simulink model "DC_Motor_WhiteBox"  (R2023b)
settings: Solver=VariableStepAuto  StartTime=0.0  StopTime=10.0  RelTol=1e-3
libraries: fl_lib x5, nesl_utility x4, ee_lib x2
settings Model: Creator=Lucas  LastModifiedBy=Lucas

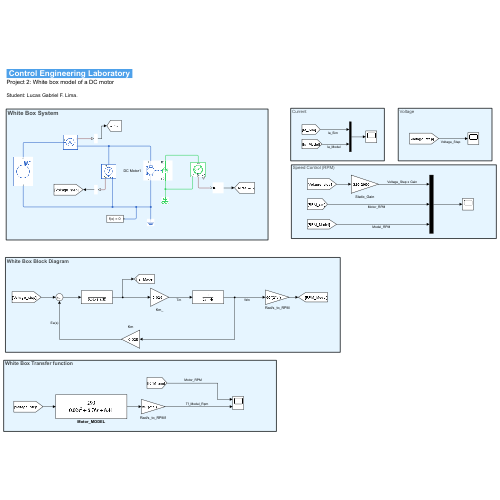
[thumbnail: Simulink's stored preview of the top-level diagram]
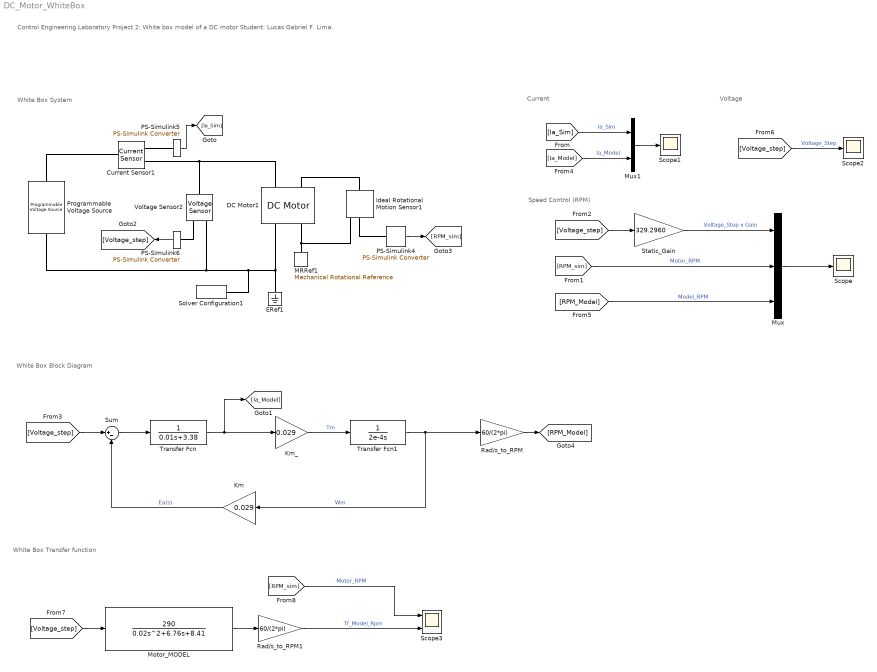
== system DC_Motor_WhiteBox ==
  note: White Box Block Diagram
  note: Speed Control (RPM)
  note: Current
  note: White Box System
  note: White Box Transfer function
  note: Control Engineering Laboratory
      | Project 2: White box model of a DC motor
      |
      | Student: Lucas Gabriel F. Lima.
  note: Voltage
  Current Sensor1 : fl_lib/Electrical/Electrical Sensors/Current Sensor
  DC Motor1 : ee_lib/Electromechanical/Brushed Motors/DC Motor  field_option=ee.enum.field_option.pm  Rf=100 Ohm  Lf=1 H  Laf=0.15 H  If0=0 A  parameterization=ee.enum.dcparam_option.circuit_param  Ra=3.38 Ohm  La=0.01 H  emf_or_torque=ee.enum.emf_or_torque.kv  Kv=0.029 V/(rad/s)  Ki=6.876e-04 N*m/A  T_stall=0.1 N*m  w_max=4000 rpm  w_rated=2500 rpm  P_rated=10 W  V_rated=12 V  lam_param=ee.enum.lam_param.damping  i_noload=0 A  V_i_noload=1.5 V  J=0.0002 kg*m^2  lam=0 N*m/(rad/s)  speed0=0 rpm  enable_fault_armature=simscape.enum.onoff.off  rev_faulted=1 / 3  G_faulted_armature=1e-5 S  fault_trigger_armature=ee.enum.faults.faultTrigger.temporal  t_fault_armature=1 s  max_permissible_current_armature=inf A  t_fail_on_current_armature=1 s  enable_fault_field=simscape.enum.onoff.off  G_faulted_field=1e-5 S  fault_trigger_field=ee.enum.faults.faultTrigger.temporal  t_fault_field=1 s  max_permissible_current_field=inf A  t_fail_on_current_field=1 s  fault_action=simscape.enum.assert.action.none  alpha=3.93e-3 1/K  Tmeas=25 degC  thermal_mass=100 J/K  initial_temperature=25 degC
  ERef1 : fl_lib/Electrical/Electrical Elements/Electrical Reference
  Ideal Rotational Motion Sensor1 : fl_lib/Mechanical/Mechanical Sensors/Ideal Rotational Motion Sensor  reference=foundation.enum.MeasurementReference.difference  acceleration_port=false  velocity_port=true  position_port=true  wrap_angle=simscape.enum.onoff.off  offset=0 deg
  Km : Gain  Gain=0.029
  Km_ : Gain  Gain=0.029
  MRRef1 : fl_lib/Mechanical/Rotational Elements/Mechanical Rotational Reference
  Motor_MODEL : TransferFcn  Numerator=[290]  Denominator=[0.02 6.76 8.41]
  Mux : Mux  Inputs=3
  Mux1 : Mux  Inputs=2
  PS-Simulink4 : nesl_utility/PS-Simulink Converter  PhysicalDomain=network_engine_domain  SubClassName=ps_output  LeftPortType=input  RightPortType=output  PseudoPeriodic=off  Frequencies=[]  VectorFormat=1-D array  Unit=rpm  AffineConversion=off
  PS-Simulink5 : nesl_utility/PS-Simulink Converter  PhysicalDomain=network_engine_domain  SubClassName=ps_output  LeftPortType=input  RightPortType=output  PseudoPeriodic=off  Frequencies=[]  VectorFormat=1-D array  Unit=A  AffineConversion=off
  PS-Simulink6 : nesl_utility/PS-Simulink Converter  PhysicalDomain=network_engine_domain  SubClassName=ps_output  LeftPortType=input  RightPortType=output  PseudoPeriodic=off  Frequencies=[]  VectorFormat=1-D array  Unit=V  AffineConversion=off
  Programmable Voltage Source : ee_lib/Sources/Programmable Voltage Source  magnitude_type=ee.enum.timechanging.constant  ac_magnitude=0 V  magn_ramp=1 V/s  magn_step=1 V  magn_modu_magn=1 V  magn_modu_freq=1 Hz  magn_t1=1 s  magn_t2=2 s  frequency_type=ee.enum.timechanging.constant  ac_frequency=60 Hz  freq_ramp=1 Hz/s  freq_step=1 Hz  freq_modu_magn=1 Hz  freq_modu_freq=1 Hz  freq_t1=1 s  freq_t2=2 s  phase_type=ee.enum.timechanging.constant  ac_shift=0 deg  phase_ramp=1 deg/s  phase_step=1 deg  phase_modu_magn=1 deg  phase_modu_freq=1 Hz  phase_t1=1 s  phase_t2=2 s  dc_type=ee.enum.timechanging.step  dc_voltage=0 V  dc_ramp=1 V/s  dc_step=1 V  dc_modu_magn=1 V  dc_modu_freq=1 Hz  dc_t1=1 s  dc_t2=10 s  harmonic_option=0  harmonic_orders=[5, 7, 11, 13]  harmonic_ratios=[.1, .1, .1, .1]  harmonic_shifts=[0, 0, 0, 0] deg  harmonic_t1=-inf s  harmonic_t2=inf s  noise_mode=0  PSD=0 V^2/Hz  repeatability=1  auto_seed=0  user_seed=0  sample_time=1e-3 s  i_specify=off  i_priority=None  i=0 A  i_nominal_specify=off  i_nominal_unit=A  i_nominal_value=1  v_specify=off  v_priority=None  v=0 V  v_nominal_specify=off  v_nominal_unit=V  v_nominal_value=1
      settings: InternalSimscapePortConfiguration="{\"Bottom\":[],\"Left\":[{\"id\":\"p\",\"label\":\"+\",\"type\":\"foundation.electrical.electrical\"}],\"Right\":[{\"id\":\"n\",\"label\":\"-\",\"type\":\"foundation.electrical.electrical\"}],\"Top\":[]}"
  Rad/s_to_RPM : Gain  Gain=60/(2*pi)
  Rad/s_to_RPM1 : Gain  Gain=60/(2*pi)
  Scope : Scope
  Scope1 : Scope
  Scope2 : Scope
  Scope3 : Scope  NumInputPorts=2
  Solver Configuration1 : nesl_utility/Solver Configuration  PhysicalDomain=network_engine_domain  SubClassName=solver  LeftPortType=input  RightPortType=generic  Tones=[]  Harmonics=[]  SimulateNoise=off  Profile=off  UseLocalSampling=off  EnableSwitchedLinearOptims=on  FrequencyDomain=off  UseCCode=off  RelTol=0.001  AbsTol=1e-06  MinStep=1e-09  ToWorkspace=off  RevertToSquareIcSolve=off  NumHomotopyIterations=100  PhasorMode=off  PhasorModeNumHarmonics=1  ConsistencySolver=NEWTON_FTOL  IndexReductionMethod=DerivativeReplacement  DoDC=off  ResidualTolerance=1e-9  ConsistencyTolSource=GLOBAL  ConsistencyAbsTol=0.001  ConsistencyRelTol=0.001  ConsistencyTolFactor=0.001  UseLocalSolver=off  LocalSolverChoice=NE_BACKWARD_EULER_ADVANCER  ResolveIndetEquations=on  FunctionEvalNumThread=1  LocalSolverSampleTime=5e-6  DoFixedCost=off  MaxNonlinIter=4  MaxModeIter=2  ComputeImpulses=off  ImpulseIterations=2  LinearAlgebra=auto  LinearAlgebraNumThread=0  EquationFormulation=NE_TIME_EF  DelaysMemoryBudget=1024  AutomaticFiltering=on  FilteringTimeConstant=0.001  PartitionStorageMethod=AS_NEEDED  PartitionMemoryBudget=1024  PartitionMethod=FAST  MultibodyUseLocalSolver=off  MultibodyLocalSolverChoice=ODE1  MultibodyLocalSolverSampleTime=0.001
  Static_Gain : Gain  Gain=329.2960
  Sum : Sum  Inputs=|+-
  Transfer Fcn : TransferFcn  Denominator=[0.01 3.38]
  Transfer Fcn1 : TransferFcn  Denominator=[2e-4 0]
  Voltage Sensor2 : fl_lib/Electrical/Electrical Sensors/Voltage Sensor
  wires:
  PS-Simulink4/1 -> [RPM_sim]
  [Ia_Sim] -> Mux1/1  "Ia_Sim"
  PS-Simulink5/1 -> [Ia_Sim]
  [Voltage_step] -> Static_Gain/1
  [RPM_sim] -> Mux/2  "Motor_RPM"
  [RPM_Model] -> Mux/3  "Model_RPM"
  Mux/1 -> Scope/1
  Transfer Fcn/1 -> Km_/1, [Ia_Model]
  [Voltage_step] -> Sum/1
  PS-Simulink6/1 -> [Voltage_step]
  Sum/1 -> Transfer Fcn/1
  Rad/s_to_RPM/1 -> [RPM_Model]
  Km/1 -> Sum/2  "Ea(s)"
  Km_/1 -> Transfer Fcn1/1  "Tm"
  Transfer Fcn1/1 -> Km/1, Rad/s_to_RPM/1  "Wm"
  [Ia_Model] -> Mux1/2  "Ia_Model"
  [Voltage_step] -> Scope2/1  "Voltage_Step"
  Mux1/1 -> Scope1/1
  Static_Gain/1 -> Mux/1  "Voltage_Step x Gain"
  [Voltage_step] -> Motor_MODEL/1
  Motor_MODEL/1 -> Rad/s_to_RPM1/1
  Rad/s_to_RPM1/1 -> Scope3/2  "Tf_Model_Rpm"
  [RPM_sim] -> Scope3/1  "Motor_RPM"
  connections:
  Programmable Voltage Source/RConn1 -- Voltage Sensor2/RConn2 -- Solver Configuration1/RConn1 -- DC Motor1/RConn1 -- ERef1/LConn1
  Current Sensor1/RConn2 -- DC Motor1/LConn1 -- Voltage Sensor2/LConn1
  MRRef1/LConn1 -- Ideal Rotational Motion Sensor1/RConn1 -- DC Motor1/RConn2
  Programmable Voltage Source/LConn1 -- Current Sensor1/LConn1
  Ideal Rotational Motion Sensor1/RConn2 -- PS-Simulink4/LConn1
  DC Motor1/LConn2 -- Ideal Rotational Motion Sensor1/LConn1
  PS-Simulink6/LConn1 -- Voltage Sensor2/RConn1
  Current Sensor1/RConn1 -- PS-Simulink5/LConn1
